simulink model "Modelo_Tanque_Controlado_2DOF"  (R2022a)
settings: Solver=FixedStepAuto  StartTime=0.0  StopTime=5000  FixedStep=1e-3  RelTol=1e-3
undefined symbols (not defined in the file or in its folder): Am, B1, Bm, R, S, Tnum, Ts
libraries: simulink x2
settings Model: Creator=User  LastModifiedBy=User
settings DebuggingCC: UnconnectedInputMsg=warning  UnconnectedOutputMsg=warning  UnconnectedLineMsg=warning
settings RTWCC: DLArmComputeVersion=19.05

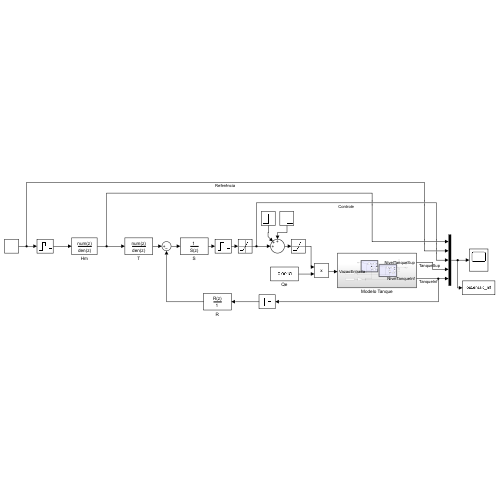
[thumbnail: Simulink's stored preview of the top-level diagram]
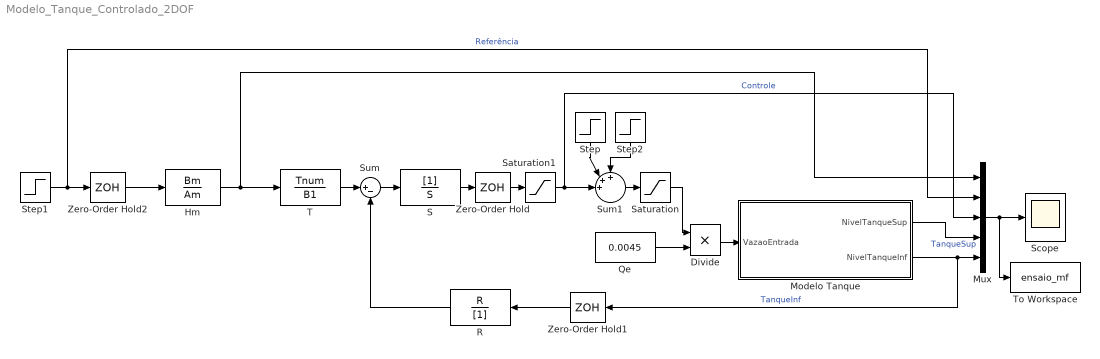
== system Modelo_Tanque_Controlado_2DOF ==
  Divide : Product  Inputs=**
  Hm : DiscreteFilter  Numerator=Bm  Denominator=Am  SampleTime=Ts
  Modelo Tanque : Subsystem
  Mux : Mux  Inputs=5
  Qe : Constant  Value=0.0045
  R : DiscreteFilter  Numerator=R  Denominator=[1]  SampleTime=Ts
  S : DiscreteFilter  Denominator=S  SampleTime=Ts
  Saturation : Saturate  UpperLimit=1  LowerLimit=0
  Saturation1 : Saturate  UpperLimit=1  LowerLimit=0
  Scope : Scope
  Step : Step  Time=2000  After=0.4  SampleTime=0
  Step1 : Step  Time=1000  Before=1.5  After=2  SampleTime=0
  Step2 : Step  Time=3000  After=-0.4  SampleTime=0
  Sum : Sum  Inputs=|+-
  Sum1 : Sum  Inputs=+++||
  T : DiscreteFilter  Numerator=Tnum  Denominator=B1  SampleTime=Ts
  To Workspace : ToWorkspace  VariableName=ensaio_mf  SaveFormat=Timeseries  SampleTime=40
  Zero-Order Hold : ZeroOrderHold  SampleTime=Ts
  Zero-Order Hold1 : ZeroOrderHold  SampleTime=Ts
  Zero-Order Hold2 : ZeroOrderHold  SampleTime=Ts
  wires:
  Qe/1 -> Divide/2
  Divide/1 -> Modelo Tanque/1(VazaoEntrada)
  Saturation/1 -> Divide/1
  Modelo Tanque/1(NivelTanqueSup) -> Mux/4  "TanqueSup"
  Modelo Tanque/2(NivelTanqueInf) -> Zero-Order Hold1/1, Mux/5  "TanqueInf"
  Mux/1 -> To Workspace/1, Scope/1
  T/1 -> Sum/1
  R/1 -> Sum/2
  Sum/1 -> S/1
  S/1 -> Zero-Order Hold/1
  Zero-Order Hold1/1 -> R/1
  Zero-Order Hold2/1 -> Hm/1
  Sum1/1 -> Saturation/1
  Step/1 -> Sum1/2
  Zero-Order Hold/1 -> Saturation1/1
  Saturation1/1 -> Sum1/3, Mux/3  "Controle"
  Step1/1 -> Mux/2, Zero-Order Hold2/1  "Referência"
  Hm/1 -> T/1, Mux/1
  Step2/1 -> Sum1/1

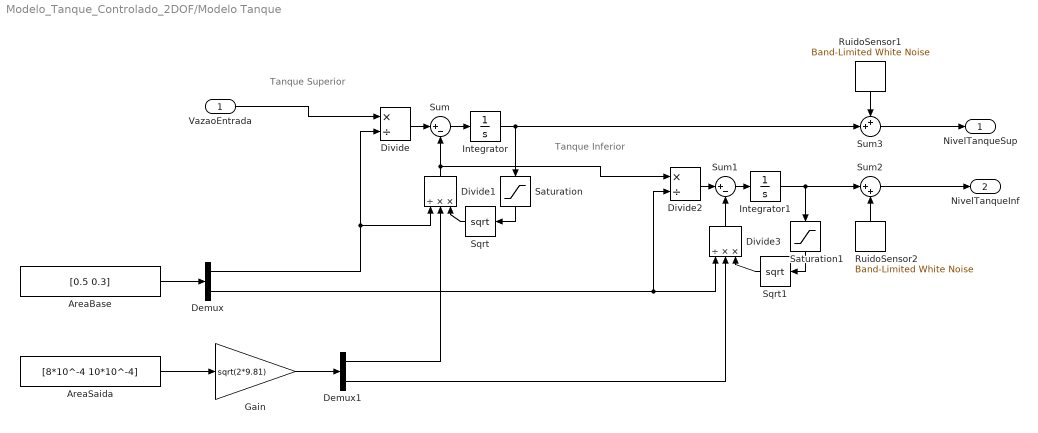
== system Modelo_Tanque_Controlado_2DOF/Modelo Tanque ==
  note: Tanque Inferior
  note: Tanque Superior
  VazaoEntrada : Inport
  AreaBase : Constant  Value=[0.5 0.3]
  AreaSaida : Constant  Value=[8*10^-4 10*10^-4]
  Demux : Demux  Outputs=2
  Demux1 : Demux  Outputs=2
  Divide : Product  Inputs=*/
  Divide1 : Product  Inputs=/**
  Divide2 : Product  Inputs=*/
  Divide3 : Product  Inputs=/**
  Gain : Gain  Gain=sqrt(2*9.81)
  Integrator : Integrator
  Integrator1 : Integrator
  RuidoSensor1 : simulink/Sources/Band-Limited White Noise  Cov=[0.00001]  Ts=1  seed=[23341]
  RuidoSensor2 : simulink/Sources/Band-Limited White Noise  Cov=[0.00001]  Ts=1  seed=[23341]
  Saturation : Saturate  UpperLimit=inf  LowerLimit=0
  Saturation1 : Saturate  UpperLimit=inf  LowerLimit=0
  Sqrt : Sqrt
  Sqrt1 : Sqrt
  Sum : Sum  Inputs=|+-
  Sum1 : Sum  Inputs=|+-
  Sum2 : Sum  Inputs=|++
  Sum3 : Sum  Inputs=++|
  NivelTanqueSup : Outport
  NivelTanqueInf : Outport  Port=2
  wires:
  AreaSaida/1 -> Gain/1
  AreaBase/1 -> Demux/1
  Gain/1 -> Demux1/1
  Sum3/1 -> NivelTanqueSup/1
  Integrator/1 -> Saturation/1, Sum3/2
  Demux/1 -> Divide/2, Divide1/1
  Divide/1 -> Sum/1
  Sum/1 -> Integrator/1
  Demux1/1 -> Divide1/2
  Sqrt/1 -> Divide1/3
  Integrator1/1 -> Sum2/1, Saturation1/1
  Demux1/2 -> Divide3/2
  Sqrt1/1 -> Divide3/3
  Divide3/1 -> Sum1/2
  Demux/2 -> Divide3/1, Divide2/2
  Sum1/1 -> Integrator1/1
  Divide2/1 -> Sum1/1
  Sum2/1 -> NivelTanqueInf/1
  RuidoSensor2/1 -> Sum2/2
  RuidoSensor1/1 -> Sum3/1
  VazaoEntrada/1 -> Divide/1
  Divide1/1 -> Divide2/1, Sum/2
  Saturation/1 -> Sqrt/1
  Saturation1/1 -> Sqrt1/1
